simulink model "vehicle_model"  (R2017a)
settings: Solver=VariableStepAuto  StartTime=0.0  StopTime=1180  MaxStep=0.01  RelTol=1e-3  EnableMultiTasking=on
values from neighbouring files (symbols this model uses):
  a = 1    [DATI_Veicolo.m]    (also in internal_permanent_magnet_motor.m = fluxM/(Ld*Inn))
  af = 1    [DATI_Veicolo.m]
  b = 1    [DATI_Veicolo.m]
  c = max(t_out)    [brushless_motor_characteristic.m]
  cd = 0.652    [DATI_Veicolo.m]
  crr_f = 0.0085    [DATI_Veicolo.m]
  crr_r = 0.0085    [DATI_Veicolo.m]
  losses_data = losses_data'    [brushless_motor_characteristic.m]
  mg = np*mh+mp+mc    (= 1772)    [DATI_Veicolo.m]
  n = max(n_out)    [brushless_motor_characteristic.m]
  n_data = [10:100:10100]    [brushless_motor_characteristic.m]
  rho = 1.2041    [DATI_Veicolo.m]
  rt = 4.3    [DATI_Veicolo.m]
  rw = (x3*25.4/1000)/2+x1*x2/100000    (= 0.3262)    [DATI_Veicolo.m]
  t_data = [1:1:max(max(t_out))]    [brushless_motor_characteristic.m]
libraries: simulink x11
settings Model: Creator=matte  LastModifiedBy=matte
settings DataIOCC: LimitDataPoints=on
settings OptimizationCC: LifeSpan=inf
settings DebuggingCC: AllowSymbolicDim=off  SFUnexpectedBacktrackingDiag=warning  SFNoUnconditionalDefaultTransitionDiag=warning  SFExecutionAtInitializationDiag=none
settings ModelReferenceCC: PropagateSignalLabelsOutOfModel=off
settings GRTTargetCC: TargetLangStandard=C89/C90 (ANSI)
settings ConfigComp: CovMetricSettings=dw  CovHtmlReporting=on  CovSaveCumulativeToWorkspaceVar=on  CovSaveSingleToWorkspaceVar=on  CovExternalEMLEnable=off

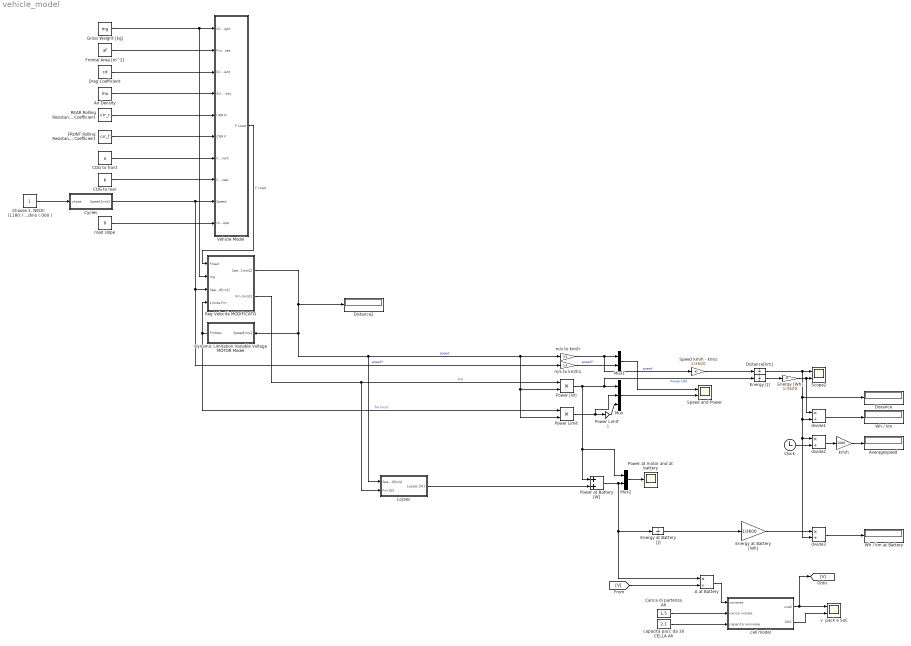
== system vehicle_model ==
  A at Battery : Product  Inputs=*/
  Air Density : Constant  Value=rho
  Averagespeed : Display
  COG to front : Constant  Value=a
  COG to rear : Constant  Value=b
  Carica di partenza Ah : Constant  Value=1.5
  "Choose 1. NEDC \t\t\t\t(1180 ) 2.Urban \t\t\t\t( 994 ) 3.Rural \t\t\t\t(1083 ) 4.MotorWay\t \t\t(1069 ) 5.Bologna Viali\t \t\t( 971 ) 6.Roma San Basilio \t\t( 522 ) 7.Gradino\t\t\t( 000 ) " : Constant
  Clock : Clock
  Cycles : Subsystem
  Distance : Display
  Distance2 : Display
  Distance[km] : Integrator
  Drag Coefficient : Constant  Value=cd
  Dynamic Limitation Variable Voltage MOTOR Model : Subsystem
  Energy [J] : Integrator
  Energy [Wh] : Gain  Gain=1/3600
  Energy at Battery [J] : Integrator
  Energy at Battery [Wh] : Gain  Gain=1/3600
  FRONT Rolling Resistance Coefficient : Constant  Value=crr_f
  Frontal Area [m^2] : Constant  Value=af
  Gross Weight [kg] : Constant  Value=mg
  Losses : Subsystem
  Mux : Mux  Inputs=3
  Mux1 : Mux  Inputs=2
  Mux2 : Mux  Inputs=2
  Power Limit : Product  Inputs=**
  Power Limit' : Gain  Gain=-1
  Power [W] : Product  Inputs=**
  Power at Battery [W] : Sum
  "Power at motor and at battery " : Scope
  REAR Rolling Resistance Coefficient : Constant  Value=crr_r
  Reg Velocità MODIFICATO : Subsystem
  Scope2 : Scope  NumInputPorts=2
  Speed and Power : Scope  NumInputPorts=2
  Speed km/h - km/s : Gain  Gain=1/3600
  Vehicle Model : Subsystem
  Wh / km : Display
  Wh / km at Battery : Display
  capacità pacc da 30 CELLA Ah : Constant  Value=2.1
  cell model : Subsystem
  divide1 : Product  Inputs=*/
  divide2 : Product  Inputs=*/
  divide3 : Product  Inputs=*/
  km/h : Gain  Gain=1000
  m/s to km/h : Gain  Gain=3.6
  m/s to km/h1 : Gain  Gain=3.6
  road slope : Constant  Value=0
  v  pack e SoC : Scope  NumInputPorts=2
  wires:
  Gross Weight [kg]/1 -> Vehicle Model/1(Gross Weight), Reg Velocità MODIFICATO/2(mg)
  Frontal Area [m^2]/1 -> Vehicle Model/2(Frontal Area)
  Drag Coefficient/1 -> Vehicle Model/3(Drag Coefficient)
  Air Density/1 -> Vehicle Model/4(Air Density)
  COG to front/1 -> Vehicle Model/7(COG front)
  COG to rear/1 -> Vehicle Model/8(COG rear)
  road slope/1 -> Vehicle Model/10("road slope ")
  REAR Rolling Resistance Coefficient/1 -> Vehicle Model/5(CRR R)
  FRONT Rolling Resistance Coefficient/1 -> Vehicle Model/6(CRR F)
  "Choose 1. NEDC \t\t\t\t(1180 ) 2.Urban \t\t\t\t( 994 ) 3.Rural \t\t\t\t(1083 ) 4.MotorWay\t \t\t(1069 ) 5.Bologna Viali\t \t\t( 971 ) 6.Roma San Basilio \t\t( 522 ) 7.Gradino\t\t\t( 000 ) "/1 -> Cycles/1(chose)
  Vehicle Model/1(F Load) -> Reg Velocità MODIFICATO/1(Fload)  "F Load"
  Reg Velocità MODIFICATO/1(Speed [m/s]2) -> Distance2/1, Dynamic Limitation Variable Voltage MOTOR Model/1(Speed[m/s]), Losses/1(Speed[m/s]), m/s to km/h/1, Power Limit/2, Power [W]/2  "speed"
  Dynamic Limitation Variable Voltage MOTOR Model/1("FmMax ") -> Reg Velocità MODIFICATO/4(Limite Fm), Power Limit/1  "fm limit"
  Reg Velocità MODIFICATO/2(Fm [m/s]2) -> Losses/2(Fm [N]), Power [W]/1  "Fm"
  Power [W]/1 -> Mux2/1, Power at Battery [W]/1, Energy [J]/1, Mux/1  "Power [W]"
  Power Limit/1 -> Mux/2, Power Limit'/1
  Power Limit'/1 -> Mux/3
  Mux/1 -> Speed and Power/2
  Energy [Wh]/1 -> divide1/1, Scope2/2
  Energy [J]/1 -> Energy [Wh]/1
  divide1/1 -> Wh / km/1
  Clock/1 -> divide2/2
  Distance[km]/1 -> divide2/1, divide3/2, divide1/2, Distance/1, Scope2/1
  divide2/1 -> km/h/1
  km/h/1 -> Averagespeed/1
  Losses/1(Losses [W]) -> Power at Battery [W]/2
  Power at Battery [W]/1 -> A at Battery/1, Energy at Battery [J]/1, Mux2/2
  Mux2/1 -> "Power at motor and at battery "/1
  Energy at Battery [J]/1 -> Energy at Battery [Wh]/1
  Energy at Battery [Wh]/1 -> divide3/1
  divide3/1 -> Wh / km at Battery/1
  Mux1/1 -> Speed and Power/1
  m/s to km/h/1 -> Mux1/1, Speed km/h - km/s/1  "speed"
  m/s to km/h1/1 -> Mux1/2  "speed*"
  Cycles/1(Speed [m/s]) -> Vehicle Model/9(Speed), Reg Velocità MODIFICATO/3(Speed[m/s]), m/s to km/h1/1  "speed*"
  A at Battery/1 -> cell model/1(corrente)
  capacità pacc da 30 CELLA Ah/1 -> cell model/3(capacità nominale)
  Carica di partenza Ah/1 -> cell model/2(carica iniziale)
  cell model/1(vcell) -> [V], v  pack e SoC/1
  cell model/2(SOC) -> v  pack e SoC/2
  [V] -> A at Battery/2
  Speed km/h - km/s/1 -> Distance[km]/1

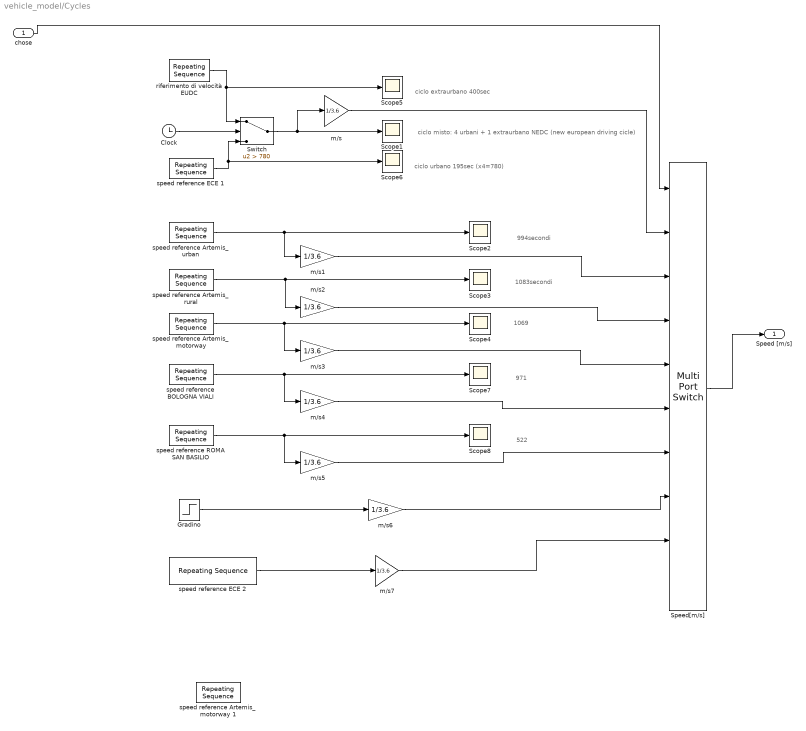
== system vehicle_model/Cycles ==
  note: 1069
  note: 522
  note: 971
  note: 1083secondi
  note: 994secondi
  note: ciclo misto: 4 urbani + 1 extraurbano NEDC (new european driving cicle)
  note: ciclo urbano 195sec (x4=780)
  note: ciclo extraurbano 400sec
  chose : Inport
  Clock : Clock
  Gradino : Step  After=130  SampleTime=0
  Scope{1..8} (8 alike) : Scope
  Speed[m/s] : MultiPortSwitch  Inputs=9
  Switch : Switch  Criteria=u2 > Threshold  Threshold=780
  m/s{,1..7} (8 alike) : Gain  Gain=1/3.6
  riferimento di velocità EUDC : simulink/Sources/Repeating Sequence  rep_seq_t=[0 20 26 37 47 61 111 119 188 201 251 286 316 336 346 362 370 380 400]  rep_seq_y=[0 0 15 35 50 70 70 50 50 70 70 100 100 120 120 80 50 0 0]
  "speed reference Artemis_motorway " : simulink/Sources/Repeating Sequence  rep_seq_t=t_artemis_motorway130  rep_seq_y=vkm_artemis_motorway130
  speed reference Artemis_motorway 1 : simulink/Sources/Repeating Sequence  rep_seq_t=t_artemis_motorway130  rep_seq_y=vkm_artemis_motorway130
  speed reference Artemis_rural : simulink/Sources/Repeating Sequence  rep_seq_t=t_artemis_rural  rep_seq_y=vkm_artemis_rural
  speed reference Artemis_urban : simulink/Sources/Repeating Sequence  rep_seq_t=t_artemis_urban  rep_seq_y=vkm_artemis_urban
  speed reference BOLOGNA VIALI : simulink/Sources/Repeating Sequence  rep_seq_t=t_bologna_viali  rep_seq_y=vkm_bologna_viali
  speed reference ECE 1 : simulink/Sources/Repeating Sequence  rep_seq_t=[0 11 15 23 28 49 55 61 85 96 117 123 134 143 155 163 178 188 195]  rep_seq_y=[0 0 15 15 0 0 15 15 32 32 0 0 15 35 50 50 35 35 0]
  speed reference ECE 2 : simulink/Sources/Repeating Sequence  rep_seq_t="[0 11 15 23 28 49 55 61 85 96 117 123 134 143 155 163 178 188 195   206   210   218   223   244   250   256   280   291   312   318   329   338   350   358   373   383   390   401   405   413   418   439   445   451   475   486   507   513   524   533   545   553   568   578   585   596   600   608   613   634   640   646   670   681   702   708   719   728   740   748   763   773   780         800         806         817         827         841         891         899         968         981        1031   1066        1096        1116        1126        1142        1150        1160        1180]"  rep_seq_y=[0 0 15 15 0 0 15 15 32 32 0 0 15 35 50 50 35 35 0 0 15 15 0 0 15 15 32 32 0 0 15 35 50 50 35 35 0 0 15 15 0 0 15 15 32 32 0 0 15 35 50 50 35 35 0 0 15 15 0 0 15 15 32 32 0 0 15 35 50 50 35 35 0 0 15 35 50 70 70 50 50 70 70 100 100 120 120 80 50 0 0]
  speed reference ROMA SAN BASILIO : simulink/Sources/Repeating Sequence  rep_seq_t=t_roma_san_basilio  rep_seq_y=vkm_roma_san_basilio
  Speed [m/s] : Outport
  wires:
  speed reference ECE 1/1 -> Scope6/1, Switch/3
  Switch/1 -> Scope1/1, m/s/1
  riferimento di velocità EUDC/1 -> Scope5/1, Switch/1
  Clock/1 -> Switch/2
  speed reference Artemis_urban/1 -> m/s1/1, Scope2/1
  m/s1/1 -> Speed[m/s]/3
  speed reference Artemis_rural/1 -> m/s2/1, Scope3/1
  m/s2/1 -> Speed[m/s]/4
  "speed reference Artemis_motorway "/1 -> m/s3/1, Scope4/1
  m/s3/1 -> Speed[m/s]/5
  speed reference BOLOGNA VIALI/1 -> m/s4/1, Scope7/1
  m/s4/1 -> Speed[m/s]/6
  speed reference ROMA SAN BASILIO/1 -> m/s5/1, Scope8/1
  m/s5/1 -> Speed[m/s]/7
  Speed[m/s]/1 -> Speed [m/s]/1
  m/s/1 -> Speed[m/s]/2
  chose/1 -> Speed[m/s]/1
  m/s6/1 -> Speed[m/s]/8
  Gradino/1 -> m/s6/1
  speed reference ECE 2/1 -> m/s7/1
  m/s7/1 -> Speed[m/s]/9

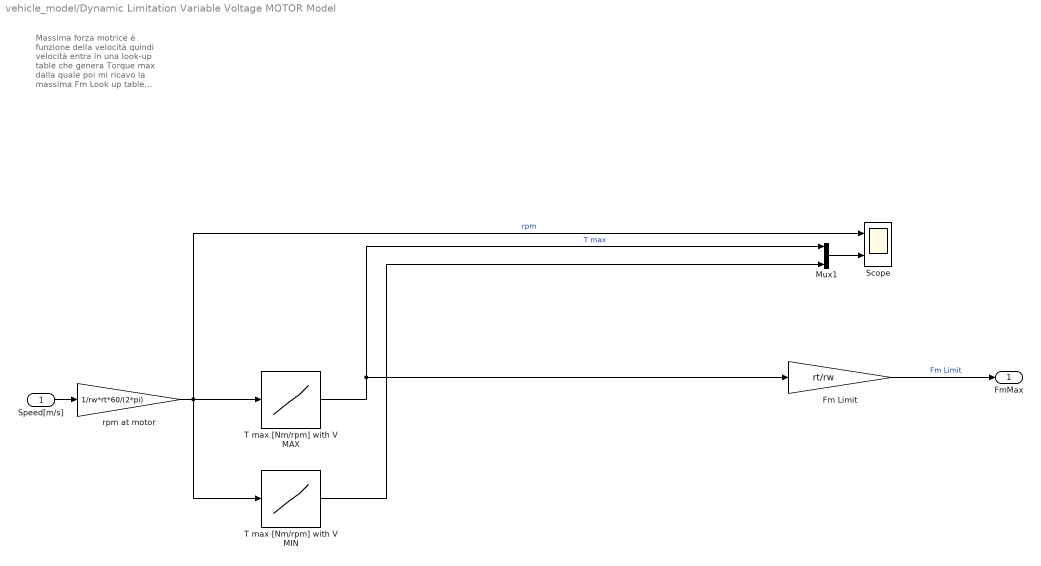
== system vehicle_model/Dynamic Limitation Variable Voltage MOTOR Model ==
  note: Massima forza motrice è funzione della velocità
      | quindi velocità entra in una look-up table che genera Torque max
      | dalla quale poi mi ricavo la massima Fm
      |
      | Look up table può essere ricavata da punti sperimentali o "fatta in casa"
      | definendo vari punti ad esempio 4
  Speed[m/s] : Inport
  Fm Limit : Gain  Gain=rt/rw
  Mux1 : Mux  Inputs=3
  Scope : Scope  NumInputPorts=2
  T max [Nm/rpm] with V MAX : Lookup_n-D  NumberOfTableDimensions=1  BreakpointsForDimension1=n  Table=c  InternalRulePriority=Speed  RndMeth=Simplest  InputSameDT=on
  T max [Nm/rpm] with V MIN : Lookup_n-D  NumberOfTableDimensions=1  BreakpointsForDimension1=n  Table=c  InternalRulePriority=Speed  RndMeth=Simplest  InputSameDT=on
  rpm at motor : Gain  Gain=1/rw*rt*60/(2*pi)
  "FmMax " : Outport
  wires:
  Speed[m/s]/1 -> rpm at motor/1
  rpm at motor/1 -> Scope/1, T max [Nm/rpm] with V MIN/1, T max [Nm/rpm] with V MAX/1  "rpm"
  Fm Limit/1 -> "FmMax "/1  "Fm Limit"
  T max [Nm/rpm] with V MIN/1 -> Mux1/3
  T max [Nm/rpm] with V MAX/1 -> Fm Limit/1, Mux1/1  "T max"
  Mux1/1 -> Scope/2

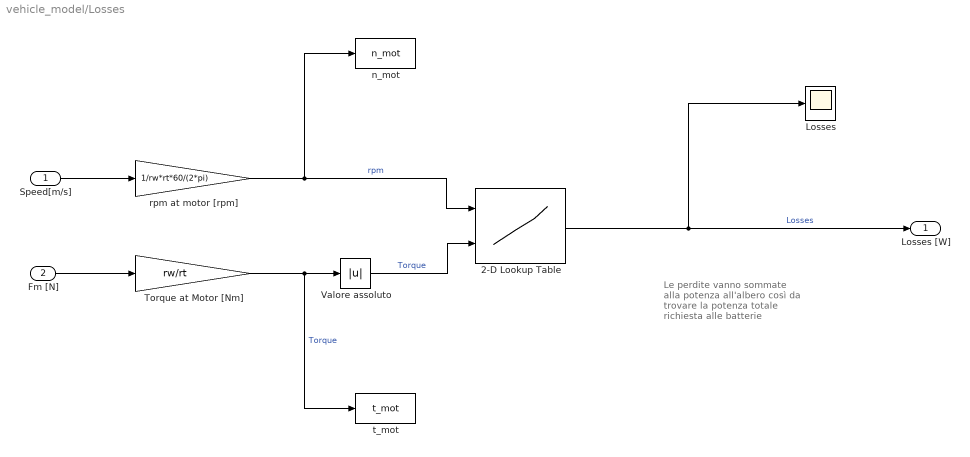
== system vehicle_model/Losses ==
  note: Le perdite vanno sommate alla potenza all'albero
      | così da trovare la potenza totale richiesta alle batterie
  Speed[m/s] : Inport
  Fm [N] : Inport  Port=2
  2-D Lookup Table : Lookup_n-D  BreakpointsForDimension1=n_data  BreakpointsForDimension2=t_data  Table=losses_data  InternalRulePriority=Speed  RndMeth=Simplest  InputSameDT=on
  Losses : Scope
  Torque at Motor [Nm] : Gain  Gain=rw/rt
  Valore assoluto : Abs
  "n_mot " : ToWorkspace  VariableName=n_mot  SampleTime=-1
  rpm at motor [rpm] : Gain  Gain=1/rw*rt*60/(2*pi)
  "t_mot " : ToWorkspace  VariableName=t_mot  SampleTime=-1
  Losses [W] : Outport
  wires:
  Speed[m/s]/1 -> rpm at motor [rpm]/1
  Fm [N]/1 -> Torque at Motor [Nm]/1
  rpm at motor [rpm]/1 -> "n_mot "/1, 2-D Lookup Table/1  "rpm"
  Torque at Motor [Nm]/1 -> Valore assoluto/1, "t_mot "/1  "Torque"
  2-D Lookup Table/1 -> Losses/1, Losses [W]/1  "Losses"
  Valore assoluto/1 -> 2-D Lookup Table/2  "Torque"

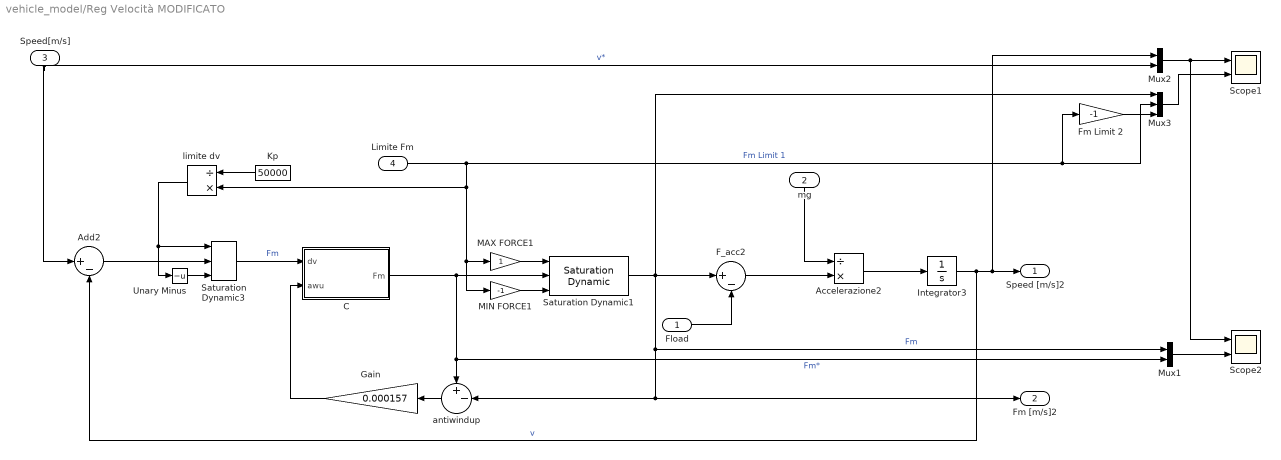
== system vehicle_model/Reg Velocità MODIFICATO ==
  Fload : Inport
  mg : Inport  Port=2
  Speed[m/s] : Inport  Port=3
  Limite Fm : Inport  Port=4
  Accelerazione2 : Product  Inputs=/*
  Add2 : Sum  Inputs=|+-
  "C " : Subsystem
  F_acc2 : Sum  Inputs=|+-
  "Fm Limit 2 " : Gain  Gain=-1
  Gain : Gain  Gain=0.000157
  Integrator3 : Integrator
  Kp : Constant  Value=50000
  MAX FORCE1 : Gain
  MIN FORCE1 : Gain  Gain=-1
  Mux1 : Mux  Inputs=2
  Mux2 : Mux  Inputs=2
  Mux3 : Mux  Inputs=3
  Saturation Dynamic1 : simulink/Discontinuities/Saturation Dynamic  OutMin=[]  OutMax=[]  OutDataTypeStr=Inherit: Same as second input  OutDataType=fixdt(1, 16)  OutScaling=2^-10  DoSatur=off
  Saturation Dynamic3 : simulink/Discontinuities/Saturation Dynamic  OutMin=[]  OutMax=[]  OutDataTypeStr=Inherit: Same as second input  OutDataType=fixdt(1, 16)  OutScaling=2^-10  DoSatur=off
  Scope1 : Scope  NumInputPorts=2
  Scope2 : Scope  NumInputPorts=2
  Unary Minus : UnaryMinus
  antiwindup : Sum  Inputs=+-|
  limite dv : Product  Inputs=/*
  Speed [m/s]2 : Outport
  Fm [m/s]2 : Outport  Port=2
  wires:
  Limite Fm/1 -> MIN FORCE1/1, MAX FORCE1/1, limite dv/2, "Fm Limit 2 "/1, Mux3/2  "Fm Limit 1"
  Integrator3/1 -> Mux2/1, Speed [m/s]2/1, Add2/2  "v"
  F_acc2/1 -> Accelerazione2/2
  Speed[m/s]/1 -> Mux2/2, Add2/1  "v*"
  mg/1 -> Accelerazione2/1
  Accelerazione2/1 -> Integrator3/1
  Fload/1 -> F_acc2/2
  Saturation Dynamic1/1 -> Mux1/1, Fm [m/s]2/1, antiwindup/2, Mux3/1, F_acc2/1  "Fm"
  limite dv/1 -> Unary Minus/1, Saturation Dynamic3/1
  Kp/1 -> limite dv/1
  Unary Minus/1 -> Saturation Dynamic3/3
  "C "/1(Fm) -> Mux1/2, antiwindup/1, Saturation Dynamic1/2  "Fm*"
  MAX FORCE1/1 -> Saturation Dynamic1/1
  MIN FORCE1/1 -> Saturation Dynamic1/3
  Mux2/1 -> Scope2/1, Scope1/1
  "Fm Limit 2 "/1 -> Mux3/3
  Mux3/1 -> Scope1/2
  antiwindup/1 -> Gain/1
  Gain/1 -> "C "/2(awu)
  Mux1/1 -> Scope2/2
  Saturation Dynamic3/1 -> "C "/1(dv)  "Fm"
  Add2/1 -> Saturation Dynamic3/2

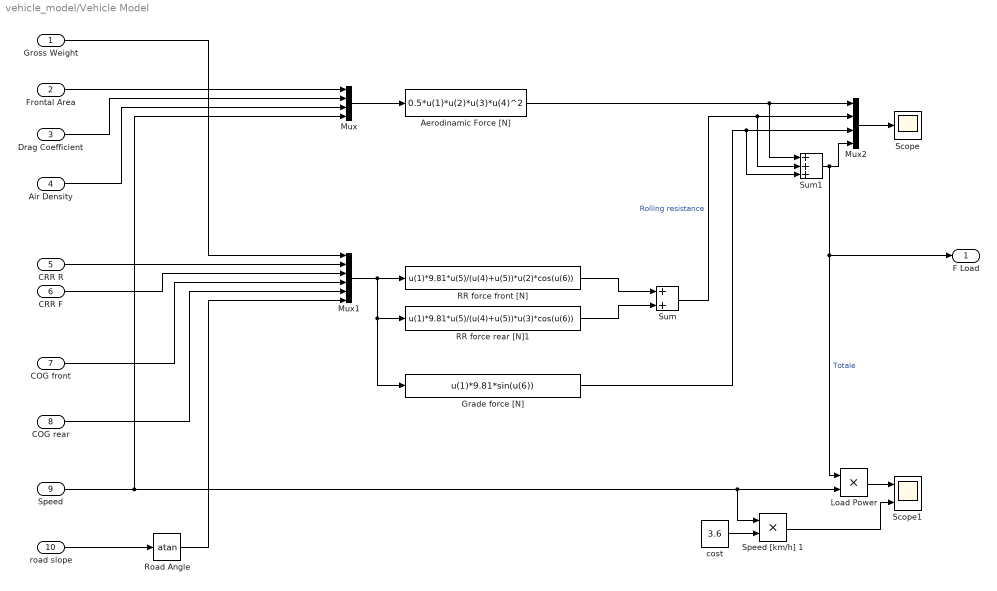
== system vehicle_model/Vehicle Model ==
  Gross Weight : Inport
  Frontal Area : Inport  Port=2
  Drag Coefficient : Inport  Port=3
  Air Density : Inport  Port=4
  CRR R : Inport  Port=5
  CRR F : Inport  Port=6
  COG front : Inport  Port=7
  COG rear : Inport  Port=8
  Speed : Inport  Port=9
  "road slope " : Inport  Port=10
  Aerodinamic Force [N] : Fcn  Expr=0.5*u(1)*u(2)*u(3)*u(4)^2
  Grade force [N] : Fcn  Expr=u(1)*9.81*sin(u(6))
  "Load Power " : Product
  Mux : Mux
  Mux1 : Mux  Inputs=6
  Mux2 : Mux
  RR force front [N] : Fcn  Expr=u(1)*9.81*u(5)/(u(4)+u(5))*u(2)*cos(u(6))
  RR force rear [N]1 : Fcn  Expr=u(1)*9.81*u(5)/(u(4)+u(5))*u(3)*cos(u(6))
  Road Angle : Trigonometry  Operator=atan
  Scope : Scope
  Scope1 : Scope  NumInputPorts=2
  Speed [km/h] 1 : Product
  Sum : Sum
  Sum1 : Sum  Inputs=+++
  "cost " : Constant  Value=3.6
  F Load : Outport
  wires:
  Drag Coefficient/1 -> Mux/2
  Speed/1 -> Mux/4, Speed [km/h] 1/1, "Load Power "/2
  Air Density/1 -> Mux/3
  "road slope "/1 -> Road Angle/1
  Frontal Area/1 -> Mux/1
  Mux1/1 -> Grade force [N]/1, RR force rear [N]1/1, RR force front [N]/1
  Gross Weight/1 -> Mux1/1
  Road Angle/1 -> Mux1/6
  RR force rear [N]1/1 -> Sum/2
  CRR R/1 -> Mux1/2
  COG front/1 -> Mux1/4
  Sum/1 -> Sum1/2, Mux2/2  "Rolling resistance"
  Sum1/1 -> F Load/1, "Load Power "/1, Mux2/4  "Totale"
  Grade force [N]/1 -> Sum1/3, Mux2/3
  COG rear/1 -> Mux1/5
  Mux/1 -> Aerodinamic Force [N]/1
  RR force front [N]/1 -> Sum/1
  CRR F/1 -> Mux1/3
  Aerodinamic Force [N]/1 -> Sum1/1, Mux2/1
  Mux2/1 -> Scope/1
  "Load Power "/1 -> Scope1/1
  "cost "/1 -> Speed [km/h] 1/2
  Speed [km/h] 1/1 -> Scope1/2

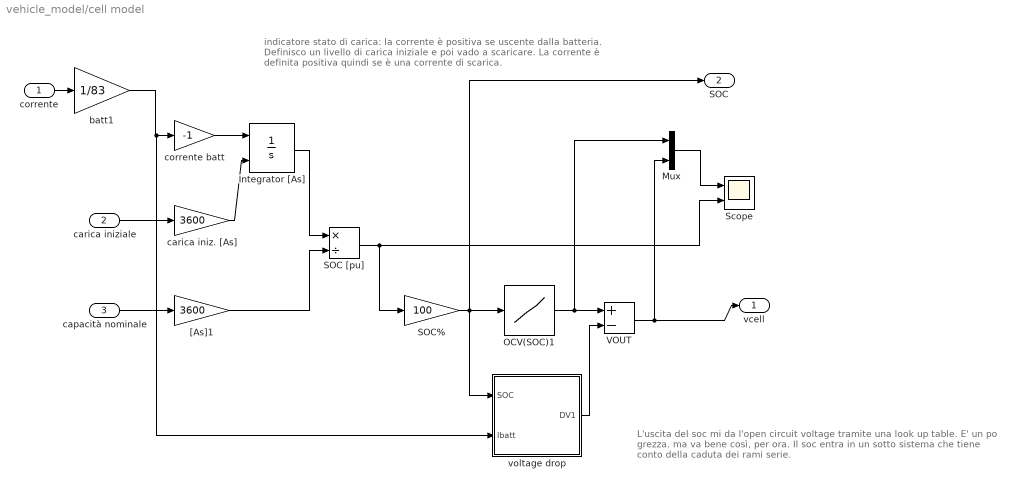
== system vehicle_model/cell model ==
  note: L'uscita del soc mi da l'open circuit voltage tramite una look up table.
      | E' un po grezza. ma va bene così, per ora. Il soc entra in un sotto sistema
      | che tiene conto della caduta dei rami serie.
  note: indicatore stato di carica: la corrente è positiva se uscente dalla batteria.
      | Definisco un livello di carica iniziale e poi vado a scaricare. La corrente è
      | definita positiva quindi se è una corrente di scarica.
  corrente : Inport
  carica iniziale : Inport  Port=2
  capacità nominale : Inport  Port=3
  Integrator [As] : Integrator  InitialConditionSource=external
  Mux : Mux  Inputs=2
  OCV(SOC)1 : Lookup  InputValues=[0 10.5 19 28.5 42 54.5 68 86 96 99 100]  Table="[235.2941  252.9412  270.5882  288.2353  294.1176  297.0588  308.8235  323.5294  335.2941  347.0588  350]"
  SOC [pu] : Product  Inputs=*/
  SOC% : Gain  Gain=100
  Scope : Scope  NumInputPorts=2
  VOUT : Sum  Inputs=+-
  "[As]1" : Gain  Gain=3600
  batt1 : Gain  Gain=1/83
  carica iniz. [As] : Gain  Gain=3600
  corrente batt : Gain  Gain=-1
  voltage drop : Subsystem  mask{rs=80e-3, rst=0.075e-3, cst=600, rlt=0.15e-3, clt=250000}
      mask prompts: rs "Series resistor RS [ohm]"; rst "short time resistance RST [ohm]"; cst "short time capacitance CST [F]"; rlt "long time resistance RLT [ohm]"; clt "long time capacitance CLT [F]"
  vcell : Outport
  SOC : Outport  Port=2
  wires:
  corrente batt/1 -> Integrator [As]/1
  carica iniz. [As]/1 -> Integrator [As]/2
  Integrator [As]/1 -> SOC [pu]/1
  "[As]1"/1 -> SOC [pu]/2
  Mux/1 -> Scope/1
  SOC [pu]/1 -> SOC%/1, Scope/2
  OCV(SOC)1/1 -> VOUT/1, Mux/1
  SOC%/1 -> OCV(SOC)1/1, SOC/1, voltage drop/1(SOC)
  voltage drop/1(DV1) -> VOUT/2
  VOUT/1 -> Mux/2, vcell/1
  carica iniziale/1 -> carica iniz. [As]/1
  capacità nominale/1 -> "[As]1"/1
  corrente/1 -> batt1/1
  batt1/1 -> voltage drop/2(Ibatt), corrente batt/1

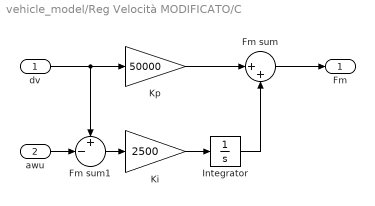
== system vehicle_model/Reg Velocità MODIFICATO/C  ==
  dv : Inport
  awu : Inport  Port=2
  Fm sum : Sum  Inputs=|++
  Fm sum1 : Sum  Inputs=+-|
  Integrator : Integrator
  Ki : Gain  Gain=2500
  Kp : Gain  Gain=50000
  Fm : Outport
  wires:
  Integrator/1 -> Fm sum/2
  Fm sum/1 -> Fm/1
  Ki/1 -> Integrator/1
  Kp/1 -> Fm sum/1
  dv/1 -> Fm sum1/1, Kp/1
  awu/1 -> Fm sum1/2
  Fm sum1/1 -> Ki/1

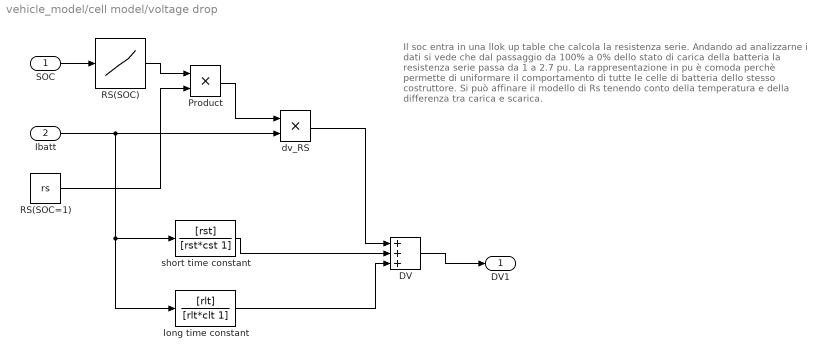
== system vehicle_model/cell model/voltage drop ==
  note: Il soc entra in una llok up table che calcola la resistenza serie. Andando
      | ad analizzarne i dati si vede che dal passaggio da 100% a 0% dello stato
      | di carica della batteria la resistenza serie passa da 1 a 2.7 pu. La rappresentazione
      | in pu è comoda perchè permette di uniformare il comportamento di tutte le celle di
      | batteria dello stesso costruttore. Si può affinare il modello di Rs tenendo conto della
      | temperatura e della differenza tra carica e scarica.
  SOC : Inport
  Ibatt : Inport  Port=2
  DV : Sum  Inputs=+++
  Product : Product  RndMeth=Zero
  RS(SOC) : Lookup  InputValues=[0 5 10 15 20 30 40 50 60 70 80 90 100]  Table=[2.7 2 1.5 1.4 1.3 1.25 1.2 1.17 1.15 1.14 1.12 1.11 1]
  RS(SOC=1) : Constant  Value=rs
  dv_RS : Product  RndMeth=Zero
  long time constant : TransferFcn  Numerator=[rlt]  Denominator=[rlt*clt 1]
  short time constant : TransferFcn  Numerator=[rst]  Denominator=[rst*cst 1]
  DV1 : Outport
  wires:
  RS(SOC)/1 -> Product/1
  RS(SOC=1)/1 -> Product/2
  Product/1 -> dv_RS/1
  SOC/1 -> RS(SOC)/1
  Ibatt/1 -> dv_RS/2, short time constant/1, long time constant/1
  short time constant/1 -> DV/2
  long time constant/1 -> DV/3
  dv_RS/1 -> DV/1
  DV/1 -> DV1/1
